simulink model "Regelstrecke_EinAusgangsLinerisierung_2024b"  (R2024b)
settings: Solver=VariableStepAuto  StartTime=0.0  StopTime=10.0  RelTol=1e-3
InitFcn:
  | % Definition der Konstanten
  | k  = 1.380649e-23;
  | e  = 1.602176634e-19;
  | T0 = 273.15; % absoluter Nullpunkt in K
  | T_C = 25; % Temperatur in °C
  | UT = k * (T0 + T_C) / e;
  | IS = 1e-8;
  | R  = 1e3;
  | L  = 100e-3;
  | C1 = 100e-9;
  | C2 = 1e-6;
  | 
  | % Werte der Stellgrößen
  | I0 = 10e-3;
  | U0 = 12;
  | 
  | syms U1_val U2_val IL_val U0_val I0_val
  | x = [U1_val, U2_val, IL_val];
  | %Zerlegung in System-, Ausgangs- und Eingangswirkung
  | f_ea = [
  |     -IS*exp(-U2_val/UT)/C1 + IL_val/C1;
  |     IL_val/C2;
  |     -U1_val/L - U2_val/L - R*IL_val/L
  | ]
  | g_ea = [
  |     0, 0;
  |     0, -1/C2;
  |     1/L, 0;
  | ]
  | g_ea_U0 = [
  |     0;
  |     0;
  |     1/L;
  | ]
  | g_ea_I0 = [
  |     0;
  |     -I0/C2;
  |     0;
  | ]
  | h_ea = U2_val %for y = xi set h_ea at position i to 1
  | 
  | %Lie-Ableitungen berechnen
  | Lf = h_ea;
  | Lf_h = Lf;
  | r = 0;
  | 
  | Lf_r = sym(zeros(10,1))
  | Lf_r(1) = Lf_h
  | 
  | 
  | while true
  |     LgLf = jacobian(Lf, x) * g_ea % x = [U1; U2; IL]
  |     if LgLf ~= 0
  |         % vermutlich notwendig, um L_f^r h anstelle von L_f^{(r-1)} h zu
  |         % erhalten
  |         Lf = jacobian(Lf, x) * f_ea
  |         Lf_h = Lf
  |         %
  |         break;
  |     end
  |     Lf = jacobian(Lf, x) * f_ea % x = [U1; U2; IL], Lf = IL/C2
  |     Lf_h = Lf
  |     Lf_r(r+2) = Lf_h
  |     r = r + 1
  | end
  | 
  | r = r + 1
  | 
  | phi = Lf_r
  | disp(Lf_r)
  | 
  | syms v
  | L_nom = v - Lf_h % letzte Lf
  | L_denom = LgLf
  | L = L_nom * pinv(L_denom)
  | 
  | alpha = LgLf
  | beta = Lf_h
  | 
  | 
  | 
  | %%%A-, B-, und C-Matrix
  | A = zeros(r);
  | for i=1:r
  |     for j=1:r
  |         if j == i+1
  |             A(i,j) = 1;
  |         end
  |     end
  | end
  | 
  | %%Oder:
  | %A = diag(ones(r-1,1), 1);
  | 
  | B = zeros(r,1);
  | B(r) = 1
  | 
  | C = zeros(1,r)
  | C(1) = 1
  | 
  | %syms U2_ref Kp
  | %v = Kp * (U2_ref - U2);
  | 
  | p = [-3, -2+1j, -2-1j];
  | 
  | G = place(A, B, p)
undefined symbols (not defined in the file or in its folder): l
settings Model: Creator=richa  LastModifiedBy=richa
settings ConfigComp: CovBoundaryAbsTol=1.0e-5

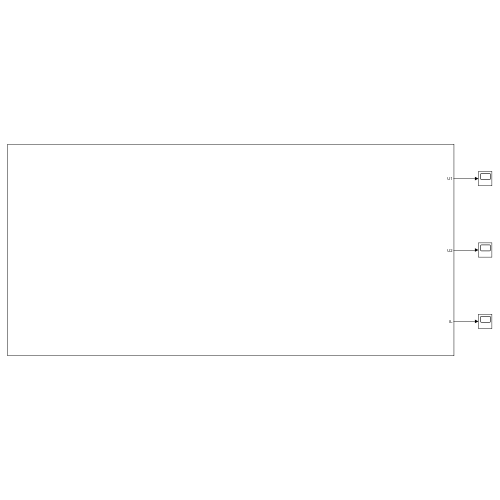
[thumbnail: Simulink's stored preview of the top-level diagram]
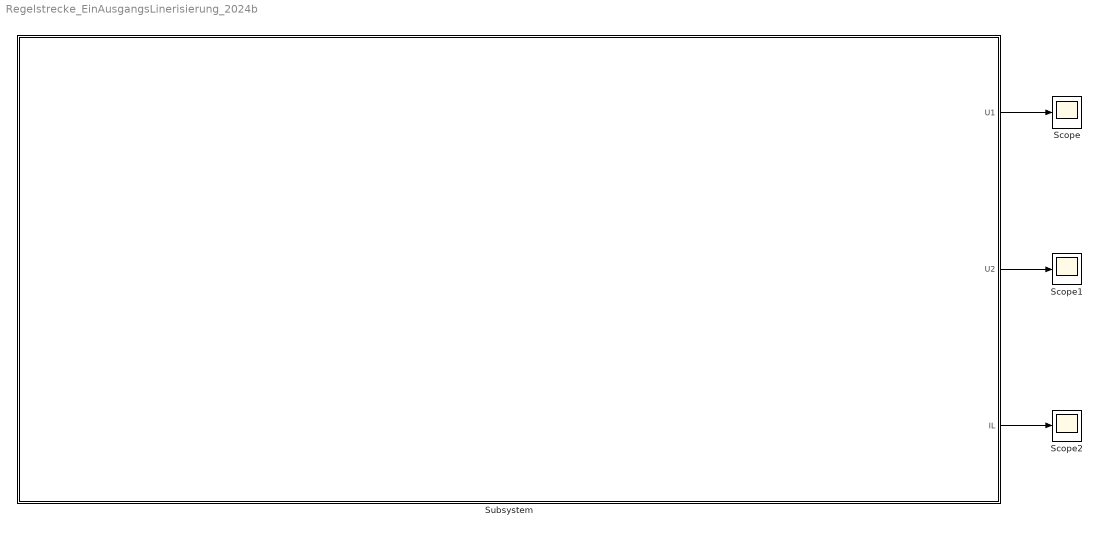
== system Regelstrecke_EinAusgangsLinerisierung_2024b ==
  Scope : Scope
  Scope1 : Scope
  Scope2 : Scope
  Subsystem : Subsystem
  wires:
  Subsystem/1(U1) -> Scope/1
  Subsystem/2(U2) -> Scope1/1
  Subsystem/3(IL) -> Scope2/1

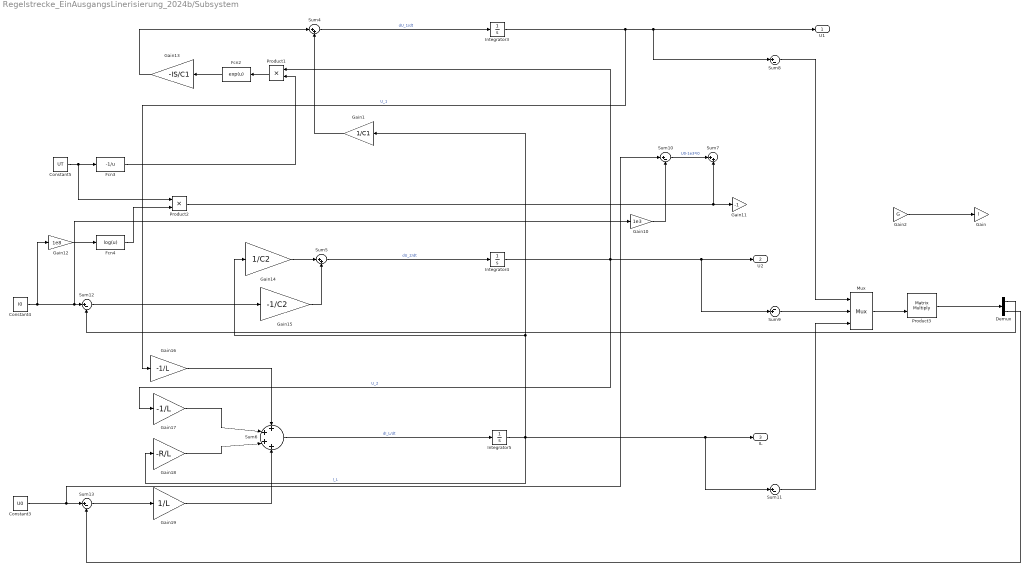
== system Regelstrecke_EinAusgangsLinerisierung_2024b/Subsystem ==
  Constant3 : Constant  Value=U0
  Constant4 : Constant  Value=I0
  Constant5 : Constant  Value=UT
  Demux : Demux  Outputs=2
  Fcn2 : Fcn  Expr=exp(u)
  Fcn3 : Fcn  Expr=-1/u
  Fcn4 : Fcn  Expr=log(u)
  Gain : Gain  Gain=l
  Gain1 : Gain  Gain=1/C1
  Gain10 : Gain  Gain=1e3
  Gain11 : Gain  Gain=-1
  Gain12 : Gain  Gain=1e8
  Gain13 : Gain  Gain=-IS/C1
  Gain14 : Gain  Gain=1/C2
  Gain15 : Gain  Gain=-1/C2
  Gain16 : Gain  Gain=-1/L
  Gain17 : Gain  Gain=-1/L
  Gain18 : Gain  Gain=-R/L
  Gain19 : Gain  Gain=1/L
  Gain2 : Gain  Gain=G
  Integrator3 : Integrator  InitialCondition=100
  Integrator4 : Integrator  InitialCondition=100
  Integrator5 : Integrator  InitialCondition=100
  Mux : Mux  Inputs=3
  Product1 : Product
  Product2 : Product
  Product3 : Product  Multiplication=Matrix(*)
  Sum{8,10..13} (5 alike) : Sum  Inputs=|+-
  Sum4 : Sum  Inputs=|++
  Sum5 : Sum  Inputs=|++
  Sum6 : Sum  Inputs=++++
  Sum7 : Sum  Inputs=|++
  Sum9 : Sum  Inputs=-+|
  U1 : Outport
  U2 : Outport  Port=2
  IL : Outport  Port=3
  wires:
  Integrator5/1 -> IL/1, Sum11/1, Gain18/1, Gain1/1, Gain14/1  "I_L"
  Integrator3/1 -> U1/1, Sum8/1, Gain16/1  "U_1"
  Product1/1 -> Fcn2/1
  Constant4/1 -> Gain12/1, Gain10/1, Sum12/1
  Product2/1 -> Gain11/1, Sum7/2
  Mux/1 -> Product3/2
  Product3/1 -> Demux/1
  Gain13/1 -> Sum4/1
  Sum10/1 -> Sum7/1  "U0-1e3*I0"
  Integrator4/1 -> U2/1, Sum9/2, Product1/1, Gain17/1  "U_2"
  Gain10/1 -> Sum10/2
  Fcn4/1 -> Product2/2
  Gain12/1 -> Fcn4/1
  Demux/1 -> Sum12/2
  Constant5/1 -> Product2/1, Fcn3/1
  Gain1/1 -> Sum4/2
  Constant3/1 -> Sum13/1, Sum10/1
  Fcn2/1 -> Gain13/1
  Gain14/1 -> Sum5/1
  Demux/2 -> Sum13/2
  Gain17/1 -> Sum6/2
  Sum12/1 -> Gain15/1
  Gain18/1 -> Sum6/3
  Gain19/1 -> Sum6/4
  Sum5/1 -> Integrator4/1  "dU_2/dt"
  Sum6/1 -> Integrator5/1  "dI_L/dt"
  Gain15/1 -> Sum5/2
  Sum13/1 -> Gain19/1
  Sum4/1 -> Integrator3/1  "dU_1/dt"
  Gain16/1 -> Sum6/1
  Fcn3/1 -> Product1/2
  Sum8/1 -> Mux/1
  Sum9/1 -> Mux/2
  Sum11/1 -> Mux/3
  Gain2/1 -> Gain/1
